simulink model "feedback_linearization_sim1"  (R2021a)
settings: Solver=VariableStepAuto  StartTime=0.0  StopTime=125  RelTol=1e-3
undefined symbols (not defined in the file): sim_output_sample_time, sim_r
settings Model: Creator=alefr  LastModifiedBy=mluser
settings DataIOCC: ReturnWorkspaceOutputs=off

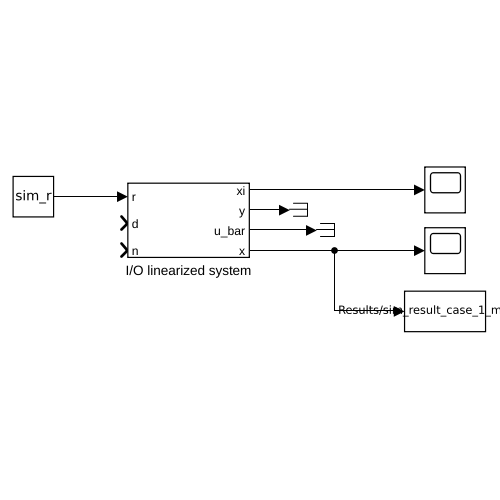
[thumbnail: Simulink's stored preview of the top-level diagram]
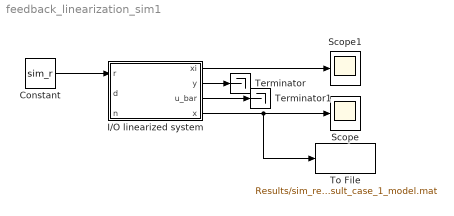
== system feedback_linearization_sim1 ==
  Constant : Constant  Value=sim_r
  I/O linearized system : Subsystem  mask{init_state_param=[8;8]}
      mask prompts: init_state_param "Initial state"
  Scope : Scope
  Scope1 : Scope
  Terminator : Terminator
  Terminator1 : Terminator
  To File : ToFile  Filename=Results/sim_result_case_1_model.mat  MatrixName=sim_result_case_1_model  SaveFormat=Timeseries  SampleTime=sim_output_sample_time
  wires:
  Constant/1 -> I/O linearized system/1(r)
  I/O linearized system/4(x) -> Scope/1, To File/1
  I/O linearized system/1(xi) -> Scope1/1
  I/O linearized system/2(y) -> Terminator/1
  I/O linearized system/3(u_bar) -> Terminator1/1

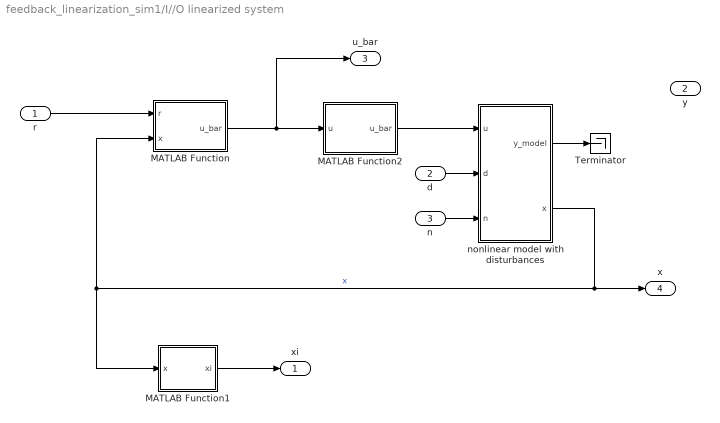
== system feedback_linearization_sim1/I//O linearized system ==
  r : Inport
  d : Inport  Port=2
  n : Inport  Port=3
  MATLAB Function : MATLAB Function  TreatAsAtomicUnit=on
  MATLAB Function1 : MATLAB Function  TreatAsAtomicUnit=on
  MATLAB Function2 : MATLAB Function  TreatAsAtomicUnit=on
  Terminator : Terminator
  nonlinear model with disturbances : Subsystem
  xi : Outport
  y : Outport  Port=2
  u_bar : Outport  Port=3
  x : Outport  Port=4
  wires:
  r/1 -> MATLAB Function/1(r)
  MATLAB Function1/1(xi) -> xi/1
  nonlinear model with disturbances/1(y_model) -> Terminator/1
  nonlinear model with disturbances/2(x) -> MATLAB Function1/1(x), MATLAB Function/2(x), x/1  "x"
  d/1 -> nonlinear model with disturbances/2(d)
  n/1 -> nonlinear model with disturbances/3(n)
  MATLAB Function2/1(u_bar) -> nonlinear model with disturbances/1(u)
  MATLAB Function/1(u_bar) -> u_bar/1, MATLAB Function2/1(u)

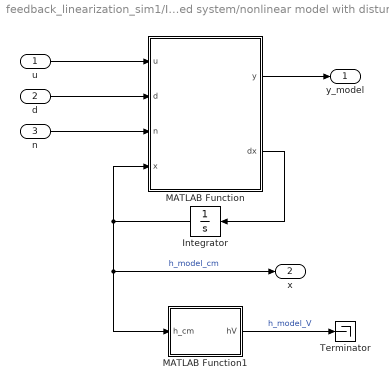
== system feedback_linearization_sim1/I//O linearized system/nonlinear model with disturbances ==
  u : Inport
  d : Inport  Port=2
  n : Inport  Port=3
  Integrator : Integrator  InitialCondition=init_state_param
  MATLAB Function : MATLAB Function  TreatAsAtomicUnit=on
  MATLAB Function1 : MATLAB Function  TreatAsAtomicUnit=on
  Terminator : Terminator
  y_model : Outport
  x : Outport  Port=2
  wires:
  MATLAB Function/1(y) -> y_model/1
  n/1 -> MATLAB Function/3(n)
  MATLAB Function1/1(hV) -> Terminator/1  "h_model_V"
  d/1 -> MATLAB Function/2(d)
  MATLAB Function/2(dx) -> Integrator/1
  Integrator/1 -> MATLAB Function/4(x), MATLAB Function1/1(h_cm), x/1  "h_model_cm"
  u/1 -> MATLAB Function/1(u)

== matlab function feedback_linearization_sim1/I//O linearized system/MATLAB Function1 ==
  data: x input; xi output
function xi = T(x)

x1 = x(1);
x2 = x(2);

xi = [x2.*7.456422751238219e-1-1.648066384406454;
    sqrt(x1.*1.962e+3+6.2784e+3).*3.841187477910597e-3-sqrt(x2.*1.962e+3+6.2784e+3).*3.841187477910597e-3];

end

== matlab function feedback_linearization_sim1/I//O linearized system/MATLAB Function2 ==
  data: u input; u_bar output
function u_bar = p(u)

u_bar = u.*9.301350851526658-u.^2.*8.172784353877083e-1+u.^3.*2.906801569971661e-2+1.237853766511371e+1;

end

== matlab function feedback_linearization_sim1/I//O linearized system/MATLAB Function ==
  data: r input; u_bar output; x input
function u_bar = k(r,x)

x1 = x(1);
x2 = x(2);

u_bar = sqrt(x1.*1.962e+3+6.2784e+3).*(r.*(3.0./8.0e+2)-x2.*2.796158531714332e-3+1.0./sqrt(x2.*1.962e+3+6.2784e+3).*(sqrt(x1.*1.962e+3+6.2784e+3).*5.151515151515152e-3-sqrt(x2.*1.962e+3+6.2784e+3).*5.151515151515152e-3).*3.768204915830296-sqrt(x1.*1.962e+3+6.2784e+3).*4.801484347388247e-4+sqrt(x2.*1.962e+3+6.2784e+3).*4.801484347388247e-4+2.559221365943785e-2).*8.757485523509194;

end

== matlab function feedback_linearization_sim1/I//O linearized system/nonlinear model with disturbances/MATLAB Function ==
  data: y output; u input; dx output; d input; n input; x input
function [y,dx] = nonlinear_model(u,d,n,x)

x1 = x(1);
x2 = x(2);

y = x2.*7.456422751238219e-1+n-1.648066384406454;

dx = [1+u.*2.818591167129287e-1-(d.*sqrt(x1.*1.962e+3+6.2784e+3))./3.3e+1-sqrt(x1.*1.962e+3+6.2784e+3).*5.151515151515152e-3-u.^2.*2.476601319356684e-2+u.^3.*8.808489605974691e-4+3.751072019731431e-1;sqrt(x1.*1.962e+3+6.2784e+3).*5.151515151515152e-3-sqrt(x2.*1.962e+3+6.2784e+3).*5.151515151515152e-3];

== matlab function feedback_linearization_sim1/I//O linearized system/nonlinear model with disturbances/MATLAB Function1 ==
  data: h_cm input; hV output
function hV = g(h_cm)

hV = h_cm*7.456422751238219e-1 - 1.648066384406454;
